simulink model "GenSync2"  (R2014b)
settings: Solver=ode45  StartTime=0.0  StopTime=35  RelTol=1e-3
values from neighbouring files (symbols this model uses):
  delta0 = double(delta)    [CalcSteady1.m]    (also in Main2.m)
  J = (1/2)*(H*S)/(ws^2)    (= 7029.15711519)    [CalcSteady1.m]    (also in CalcSteady2.m; Main.m = 3.75; Main2.m = 18500)
  Ld = 7e-3    (= 0.007)    [CalcSteady1.m]    (also in CalcSteady2.m; Main.m; Main2.m; SolverODE.m)
  Lf = 7.384e-3    (= 0.007384)    [CalcSteady1.m]    (also in CalcSteady2.m; Main.m; Main2.m; SolverODE.m)
  Lm = 6.656e-3    (= 0.006656)    [CalcSteady1.m]    (also in CalcSteady2.m; Main.m; Main2.m; SolverODE.m)
  Lq = 5.61e-3    (= 0.00561)    [CalcSteady1.m]    (also in CalcSteady2.m; Main.m; Main2.m; SolverODE.m)
  phi_D0 = double(phi_d)    [CalcSteady1.m]    (also in Main2.m)
  phi_F0 = double(phi_f)    [CalcSteady1.m]    (also in Main2.m)
  phi_Q0 = double(phi_q)    [CalcSteady1.m]    (also in Main2.m)
  Rf = 0.985e-3    (= 0.000985)    [CalcSteady1.m]    (also in CalcSteady2.m; Main.m; Main2.m; SolverODE.m)
  Rs = 1.6e-3    (= 0.0016)    [CalcSteady1.m]    (also in CalcSteady2.m; Main.m; Main2.m; SolverODE.m)
  Tm0 = double(Tm)    [CalcSteady1.m]    (also in Main.m = Tm; Main2.m)
  Vf = Rf*If    [CalcSteady1.m]    (also in CalcSteady2.m; Main.m = double(Rf*If); Main2.m = double(Rf*If); SolverODE.m = Vf0)
  Vrms = 20e3    (= 20000)    [CalcSteady1.m]    (also in Main.m = 22000; Main2.m; SolverODE.m = 22000)
  Wm0 = double(ws)    [CalcSteady1.m]    (also in Main2.m)
  ws = 2*pi*50    (= 314.159265359)    [CalcSteady1.m]    (also in CalcSteady2.m; Main.m; Main2.m; SolverODE.m)
settings Model: Creator=Eduardo Montilva  LastModifiedBy=Eduardo Montilva

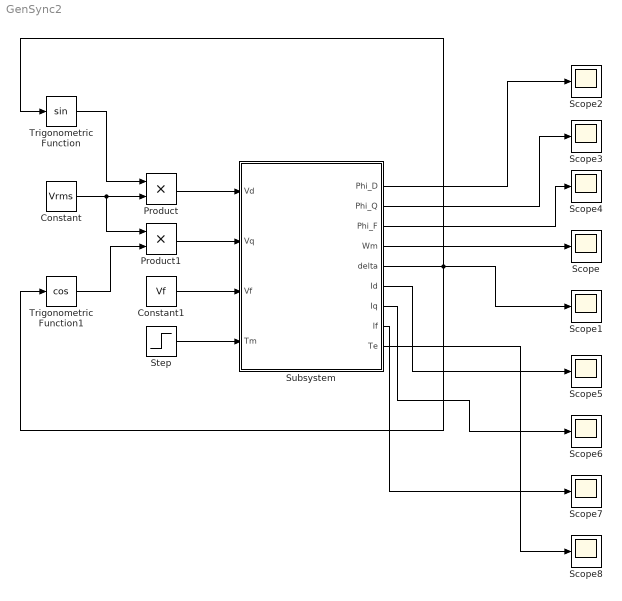
== system GenSync2 ==
  Constant : Constant  Value=Vrms
  Constant1 : Constant  Value=Vf
  Product : Product
  Product1 : Product
  Scope{,1..8} (9 alike) : Scope
      Scope settings: YMin=0  YMax=5000
      Scope2 settings: YMin=0  YMax=5000  SaveName=ScopeData2
      Scope3 settings: YMin=0  YMax=5000  SaveName=ScopeData3
      Scope4 settings: YMin=0  YMax=5000  SaveName=ScopeData4
      Scope5 settings: SaveName=ScopeData5
      Scope6 settings: SaveName=ScopeData6
      Scope7 settings: SaveName=ScopeData7
      Scope8 settings: YMin=-3e+06  YMax=3e+06  SaveName=ScopeData8
  Step : Step  Before=Tm0  After=1.7*Tm0  SampleTime=0
  Subsystem : Subsystem
  Trigonometric Function : Trigonometry
  Trigonometric Function1 : Trigonometry  Operator=cos
  wires:
  Constant/1 -> Product1/1, Product/2
  Trigonometric Function/1 -> Product/1
  Product/1 -> Subsystem/1(Vd)
  Product1/1 -> Subsystem/2(Vq)
  Trigonometric Function1/1 -> Product1/2
  Constant1/1 -> Subsystem/3(Vf)
  Step/1 -> Subsystem/4(Tm)
  Subsystem/4(Wm) -> Scope/1
  Subsystem/5(delta) -> Scope1/1, Trigonometric Function1/1, Trigonometric Function/1
  Subsystem/1(Phi_D) -> Scope2/1
  Subsystem/2(Phi_Q) -> Scope3/1
  Subsystem/3(Phi_F) -> Scope4/1
  Subsystem/6(Id) -> Scope5/1
  Subsystem/7(Iq) -> Scope6/1
  Subsystem/8(If) -> Scope7/1
  Subsystem/9(Te) -> Scope8/1

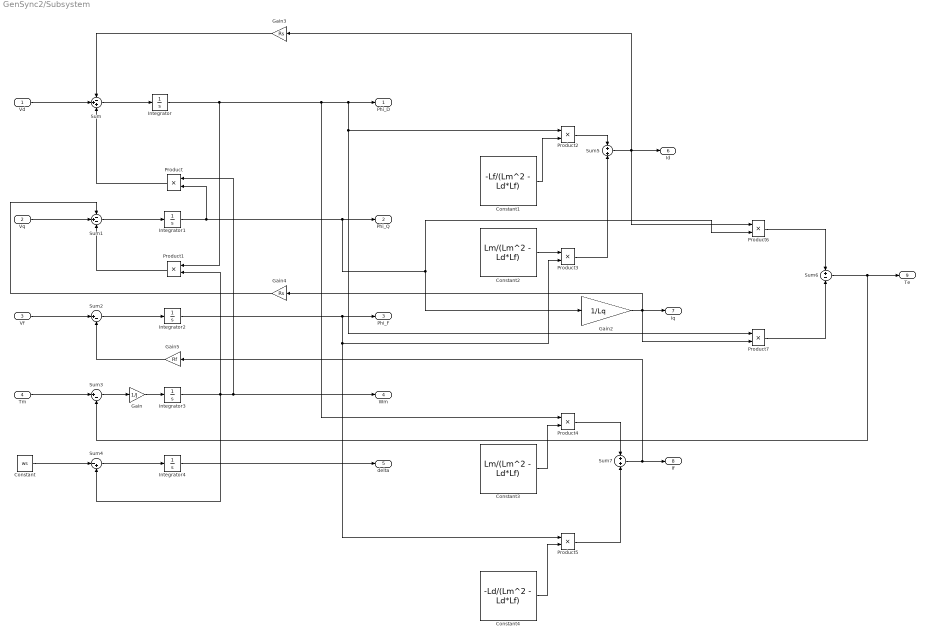
== system GenSync2/Subsystem ==
  Vd : Inport
  Vq : Inport  Port=2
  Vf : Inport  Port=3
  Tm : Inport  Port=4
  Constant : Constant  Value=ws
  Constant1 : Constant  Value=-Lf/(Lm^2 - Ld*Lf)
  Constant2 : Constant  Value=Lm/(Lm^2 - Ld*Lf)
  Constant3 : Constant  Value=Lm/(Lm^2 - Ld*Lf)
  Constant4 : Constant  Value=-Ld/(Lm^2 - Ld*Lf)
  Gain : Gain  Gain=1/J
  Gain2 : Gain  Gain=1/Lq
  Gain3 : Gain  Gain=Rs
  Gain4 : Gain  Gain=Rs
  Gain5 : Gain  Gain=Rf
  Integrator : Integrator  InitialCondition=phi_D0
  Integrator1 : Integrator  InitialCondition=phi_Q0
  Integrator2 : Integrator  InitialCondition=phi_F0
  Integrator3 : Integrator  InitialCondition=Wm0
  Integrator4 : Integrator  InitialCondition=delta0
  Product{,1..7} (8 alike) : Product
  Sum : Sum  Inputs=-++
  Sum1 : Sum  Inputs=-+-
  Sum2 : Sum  Inputs=|+-
  Sum3 : Sum  Inputs=|+-
  Sum4 : Sum  Inputs=|-+
  Sum5 : Sum
  Sum6 : Sum  Inputs=+-
  Sum7 : Sum
  Phi_D : Outport
  Phi_Q : Outport  Port=2
  Phi_F : Outport  Port=3
  Wm : Outport  Port=4
  delta : Outport  Port=5
  Id : Outport  Port=6
  Iq : Outport  Port=7
  If : Outport  Port=8
  Te : Outport  Port=9
  wires:
  Sum7/1 -> If/1, Gain5/1
  Constant/1 -> Sum4/1
  Sum2/1 -> Integrator2/1
  Integrator2/1 -> Phi_F/1, Product5/1, Product3/2
  Vd/1 -> Sum/2
  Integrator4/1 -> delta/1
  Sum4/1 -> Integrator4/1
  Sum3/1 -> Gain/1
  Sum1/1 -> Integrator1/1
  Integrator1/1 -> Product/2, Phi_Q/1, Product6/2, Gain2/1
  Vq/1 -> Sum1/2
  Integrator3/1 -> Sum4/2, Product1/2, Wm/1, Product/1
  Gain/1 -> Integrator3/1
  Product/1 -> Sum/3
  Product3/1 -> Sum5/2
  Sum/1 -> Integrator/1
  Sum5/1 -> Id/1, Product6/1, Gain3/1
  Constant1/1 -> Product2/2
  Sum6/1 -> Te/1, Sum3/2
  Gain3/1 -> Sum/1
  Vf/1 -> Sum2/1
  Gain4/1 -> Sum1/1
  Gain5/1 -> Sum2/2
  Tm/1 -> Sum3/1
  Constant2/1 -> Product3/1
  Integrator/1 -> Product1/1, Product4/1, Phi_D/1, Product7/1, Product2/1
  Constant4/1 -> Product5/2
  Product4/1 -> Sum7/1
  Product7/1 -> Sum6/2
  Product5/1 -> Sum7/2
  Product6/1 -> Sum6/1
  Product2/1 -> Sum5/1
  Constant3/1 -> Product4/2
  Gain2/1 -> Iq/1, Product7/2, Gain4/1
  Product1/1 -> Sum1/3
